simulink model "SimpleBEV3"  (R2026a)
settings: Solver=daessc  StopTime=150
libraries: fl_lib x5, nesl_utility x3, sdl_lib x2
settings Model: Creator=isaacito  LastModifiedBy=isaacito
settings SimscapeCC: SimscapeLogSimulationStatistics=on  SimscapeLogLimitData=off

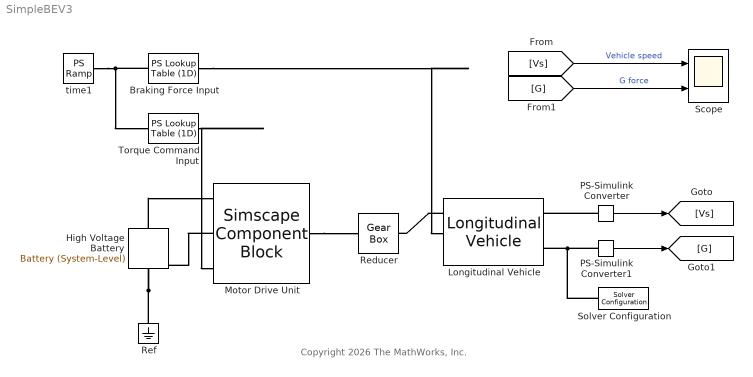
== system SimpleBEV3 ==
  note: Copyright 2026 The MathWorks, Inc.
  Braking Force Input : fl_lib/Physical Signals/Lookup Tables/PS Lookup Table (1D)  x=[0, 1, 2, 3, 4, 5] s  f=[8 8 8 0 0 0] kN  interp_method=simscape.enum.interpolation.smooth  extrap_method=simscape.enum.extrapolation.nearest
  High Voltage Battery : sdl_lib/Sources/Battery (System-Level)  Vnom=340 V  R1=0.01 Ohm  prm_AH=sdl.enum.InfiniteFinite.Infinite  AH=50 A*hr  V1=11.5 V  AH1=25 A*hr  prm_R2=sdl.enum.DisabledEnabled.Disabled  R2=2000 Ohm  thermal_port=simscape.enum.thermaleffects.omit  thermal_mass=30000 J/K  i_specify=off  i_priority=None  i=0 A  i_nominal_specify=off  i_nominal_value=1  i_nominal_unit=A  v_specify=off  v_priority=None  v=0 V  v_nominal_specify=off  v_nominal_value=1  v_nominal_unit=V  charge_specify=off  charge_priority=High  charge=50 A*hr  charge_nominal_specify=off  charge_nominal_value=1  charge_nominal_unit=A*hr  temperature_specify=off  temperature_priority=High  temperature=300 K  temperature_nominal_specify=off  temperature_nominal_value=1  temperature_nominal_unit=K
      settings: AttributesFormatString=%<Vnom> (%<Vnom_unit>)
  Longitudinal Vehicle : sdl_lib/Tires & Vehicles/Longitudinal Vehicle  vehParamType=sdl.enum.VehicleParameterizationType.Regular  M_vehicle=2200 kg  R_tireroll=0.36 m  C_tireroll=0.014  C_airdrag=0.37  A_front=2.5 m^2  A_rl=120 N  B_rl=1.8 N*s/m  C_rl=0.389 N*s^2/m^2  g=9.81 m/s^2  V_1=0.1 m/s  w_1=0.1 rad/s  ShowBrakeIn=true  ShowSlopeIn=true  SlopeInputType=sdl.enum.VehicleLongitudinalRoadSlopeInputType.Angle  ShowWindIn=false  ShowGOut=true  air_density=1.184 kg/m^3  V_x_specify=off  V_x_priority=High  V_x=0 m/s  V_x_nominal_specify=off  V_x_nominal_value=1  V_x_nominal_unit=m/s  trq_specify=off  trq_priority=None  trq=0 N*m  trq_nominal_specify=off  trq_nominal_value=1  trq_nominal_unit=N*m  w_specify=off  w_priority=None  w=0 rad/s  w_nominal_specify=off  w_nominal_value=1  w_nominal_unit=rad/s
  Motor Drive Unit : SimscapeComponentBlock  SourceFile=IdealMotorDrive  ComponentPath=IdealMotorDrive  ComponentVariants="[\"IdealMotorDrive\"]"  ComponentVariantNames="[\"IdealMotorDrive\"]"  ClassName=IdealMotorDrive  SchemaVersion=1  torque_max=160 N*m  power_max=90 kW  Tc=0.02 s  J_rotor=5*0.01^2 kg*m^2  k_fric=1e-5 N*m*s/rad  w_specify=off  w_priority=High  w=0 rpm  w_nominal_specify=off  w_nominal_value=1  w_nominal_unit=rpm
      settings: CopyFcn=simscape.sscblock.internal.componentBlockCallback(gcbh,'COPY')  PreCopyFcn=simscape.sscblock.internal.componentBlockCallback(gcbh,'PRECOPY')  PreDeleteFcn=simscape.sscblock.internal.componentBlockCallback(gcbh,'PREDELETE')
      mask Type: Ideal Motor Drive Unit
  PS-Simulink Converter : nesl_utility/PS-Simulink Converter  PhysicalDomain=network_engine_domain  SubClassName=ps_output  LeftPortType=input  RightPortType=output  PseudoPeriodic=off  Frequencies=[]  VectorFormat=inherit  Unit=km/hr  AffineConversion=off
  PS-Simulink Converter1 : nesl_utility/PS-Simulink Converter  PhysicalDomain=network_engine_domain  SubClassName=ps_output  LeftPortType=input  RightPortType=output  PseudoPeriodic=off  Frequencies=[]  VectorFormat=inherit  Unit=1  AffineConversion=off
  Reducer : fl_lib/Mechanical/Mechanisms/Gear Box  ratio=9.1  t_in_specify=off  t_in_priority=None  t_in=0 N*m  t_in_nominal_specify=off  t_in_nominal_value=1  t_in_nominal_unit=N*m  t_out_specify=off  t_out_priority=None  t_out=0 N*m  t_out_nominal_specify=off  t_out_nominal_value=1  t_out_nominal_unit=N*m
      settings: AttributesFormatString=%<ratio>
  Ref : fl_lib/Electrical/Electrical Elements/Electrical Reference
  Scope : Scope  NumInputPorts=2
      settings: ActiveDisplayYMinimum=-21.510754134953054  ActiveDisplayYMaximum=193.59678721457752
  Solver Configuration : nesl_utility/Solver Configuration  PhysicalDomain=network_engine_domain  SubClassName=solver  LeftPortType=input  RightPortType=generic  Tones=[]  Harmonics=[]  SimulateNoise=off  Profile=off  UseLocalSampling=off  EnableSwitchedLinearOptims=on  FrequencyDomain=off  UseCCode=off  RelTol=0.001  AbsTol=0.001  MinStep=1e-09  ToWorkspace=off  RevertToSquareIcSolve=off  NumHomotopyIterations=100  PhasorMode=off  PhasorModeNumHarmonics=1  ConsistencySolver=NEWTON_XTOL_AFTER_FTOL  CanonicalOrdering=CANONICAL  OptimizeIntermediates=OPTIMIZED  IndexReductionMethod=DerivativeReplacement  DoDC=off  ResidualTolerance=1e-09  ConsistencyTolSource=GLOBAL  ConsistencyAbsTol=0.001  ConsistencyRelTol=0.001  ConsistencyTolFactor=0.001  UseLocalSolver=off  LocalSolverChoice=NE_BACKWARD_EULER_ADVANCER  ResolveIndetEquations=on  FunctionEvalNumThread=1  LocalSolverSampleTime=0.001  DoFixedCost=off  MaxNonlinIter=3  MaxModeIter=2  ComputeImpulses=off  ImpulseIterations=2  LinearAlgebra=auto  LinearAlgebraNumThread=0  EquationFormulation=NE_TIME_EF  DelaysMemoryBudget=1024  AutomaticFiltering=on  FilteringTimeConstant=0.001  PartitionStorageMethod=AS_NEEDED  PartitionMemoryBudget=1024  PartitionMethod=ROBUST  MultibodyUseLocalSolver=off  MultibodyLocalSolverChoice=ODE1  MultibodyLocalSolverSampleTime=0.001
      settings: AttributesFormatString=Local solver: %<UseLocalSolver>
  Torque Command Input : fl_lib/Physical Signals/Lookup Tables/PS Lookup Table (1D)  x=[0 1 3, 4 5 75, 80 100 120, 122 130 200] s  f=[0 0 0 70 70 70 120 120 120 70 70 70] N*m  interp_method=simscape.enum.interpolation.smooth  extrap_method=simscape.enum.extrapolation.nearest
  time1 : fl_lib/Physical Signals/Sources/PS Ramp  slope=1  start_time=0 s  initial_output=0 s  ZeroCross=false
  wires:
  PS-Simulink Converter/1 -> [Vs]
  PS-Simulink Converter1/1 -> [G]
  [Vs] -> Scope/1  "Vehicle speed"
  [G] -> Scope/2  "G force"
  connections:
  time1/RConn1 -- Braking Force Input/LConn1 -- Torque Command Input/LConn1
  Longitudinal Vehicle/LConn1 -- Reducer/RConn1
  PS-Simulink Converter/LConn1 -- Longitudinal Vehicle/RConn1
  PS-Simulink Converter1/LConn1 -- Solver Configuration/RConn1 -- Longitudinal Vehicle/RConn2
  Braking Force Input/RConn1 -- Longitudinal Vehicle/LConn2
  Ref/LConn1 -- Motor Drive Unit/LConn2 -- High Voltage Battery/RConn1
  Motor Drive Unit/RConn1 -- Reducer/LConn1
  High Voltage Battery/LConn1 -- Motor Drive Unit/LConn1
  Torque Command Input/RConn1 -- Motor Drive Unit/LConn3
